simulink model "QD2_IOCheck_2021b"  (R2021b)
settings: Solver=ode2  StartTime=0.0  StopTime=inf  FixedStep=1/1000  RelTol=1e-3  EnableMultiTasking=on
undefined symbols (not defined in the file): HIL, qc_get_step_size
libraries: quarc_library x32, simulink_extras x8, simulink x7
settings Model: DataTypeOverride=Double  MinMaxOverflowLogging=ForceOff  SimulationMode=external  ExtModeTrigElement=1  ExtModeTrigDuration=10000  ExtModeTrigLevel=0.400000  Creator=dmadill  LastModifiedBy=AVRS_ADMIN
settings SolverCC: AlgebraicLoopSolver=TrustRegion  PositivePriorityOrder=on
settings DataIOCC: ReturnWorkspaceOutputs=off
settings DebuggingCC: SFMachineParentedDataDiag=warning  ArithmeticOperatorsInVariantConditions=warning
settings HardwareCC: ProdBitPerLong=64  ProdLargestAtomicInteger=LongLong  ProdLargestAtomicFloat=Double  ProdLongLongMode=on  ProdHWDeviceType=ARM Compatible->ARM 64-bit (LP64)
settings SFSimCC: SimUseLocalCustomCode=off  CustomCodeUndefinedFunction=UseInterfaceOnly
settings RTWCC: Description=QUARC Linux QDrone2 Target Using Toolchain  SystemTargetFile=quarc_linux_qdrone2.tlc  RTWUseLocalCustomCode=off  Toolchain=QUARC linux_qdrone2 | gmake (64-bit Windows)  BuildConfiguration=Faster Runs
settings CodeAppCC: StateflowObjectComments=on
settings STFCustomTargetCC: ConcurrentExecutionCompliant=on  UseToolchainInfoCompliant=on  SystemTargetFile=quarc_linux_qdrone2.tlc
settings GRTTargetCC: TargetLangStandard=C89/C90 (ANSI)  ParMdlRefBuildCompliant=off  CompOptLevelCompliant=off  CombineOutputUpdateFcns=off  MatFileLogging=off  CPPClassGenCompliant=off  GRTInterface=on  ExtMode=on  ExtModeMexFile=quarc_comm  ExtModeMexArgs='-w -d /tmp -uri %u','tcpip://192.168.2.d:17001'
settings ConfigComp: CovMetricSettings=dswe

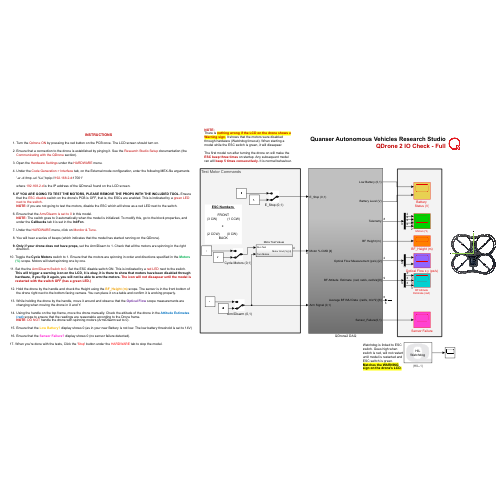
[thumbnail: Simulink's stored preview of the top-level diagram]
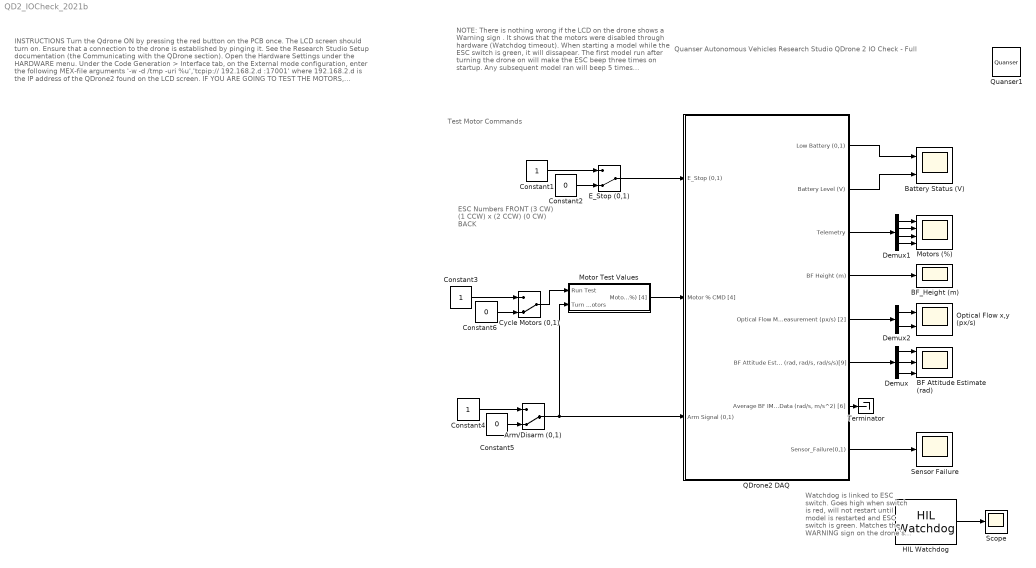
== system QD2_IOCheck_2021b ==
  note: Watchdog is linked to ESC switch. Goes high when switch is red, will not restart until model is restarted and ESC switch is green.
      | Matches the WARNING sign on the drone's LCD.
  note: Test Motor Commands
  note: Quanser Autonomous Vehicles Research Studio
      | QDrone 2 IO Check - Full
  note: ESC Numbers
      |
      | FRONT
      | (3 CW) (1 CCW)
      |
      | x
      |
      | (2 CCW) (0 CW)
      | BACK
  note: INSTRUCTIONS
      |
      | Turn the Qdrone ON by pressing the red button on the PCB once. The LCD screen should turn on.
      |
      | Ensure that a connection to the drone is established by pinging it. See the Research Studio Setup documentation (the Communicating with the QDrone section).
      |
      | Open the Hardware Settings under the HARDWARE menu.
      |
      | Under the Code Generation > Interface tab, on the External mode configuration, enter the following MEX-file arguments
      |
      | '-w -d /tmp -uri %u','tcpip:// 192.168.2.d :17001'
      |
      | where 192.168.2.d is the IP address of the QDrone2 found on the LCD screen.
      |
      | IF YOU ARE GOING TO TEST THE MOTORS, PLEASE REMOVE THE PROPS WITH THE INCLUDED TOOL. Ensure that the ESC disable switch on the drone's PCB is OFF, that is, the ESCs are enabled. This is indicated by a green LED next to the switch .
      | NOTE: if you are not going to test the motors, disable the ESC which will show as a red LED next to the switch.
      |
      | Ensure that the Arm/Disarm is set to 0 in this model.
      | NOTE: The switch goes to 0 automatically when the model is initialized. To modify this, go to the block properties, and under the Callbacks tab it is set in the InitFcn .
      |
      | Under the HARDWARE menu, click on Monitor & Tune .
      |
      | You will hear a series of beeps (which indicates that the model has started running on the QDrone).
      |
      | Only if your drone does not have props, set the Arm/Disarn to 1. Check that all the motors are spinning in the right direction.
      |
      | Toggle the Cycle Motors switch to 1. Ensure that the motors are spinning in order and directions specified in the Motors (%) scope. Motors will start spinning one by one.
      |
      | Set the the Arm/Disarm Switch to 0. Set the ESC disable switch ON. This is indicated by a red LED next to the switch. This will trigger a warning icon on the LCD, it is okay, it is there to show that motors have been disabled through hardware, if you flip it again, you will not be able to arm the motors. The icon will not dissapear until the model is restarted with the switch OFF (has a green LED.)
      |
      | Hold the drone by the handle and check the Height using the BF_Height (m) scope. The sensor is in the front bottom of the drone right next to the bottom facing camera. You can place it on a table and confirm it is working properly.
      |
      | While holding the drone by the handle, move it around and observe that the Optical Flow scope measurements are changing when moving the drone in X and Y.
      |
      | Using the handle on the top frame, move the drone manually. Check the attitude of the drone in the Attitude Estimates (rad) scope to ensure that the readings are reasonable according to the Drone frame.
      | NOTE : DO NOT handle the drone with spinning motors (Arm/Disarm set to 0).
      |
      | Ensure that the Low Battery? display shows 0 (as in your new Battery is not low. The low battery threshold is set to 14V)
      |
      | Ensure that the Sensor Failure? display shows 0 (no sensor failure detected).
      |
      | When you're done with the tests, Click the ' Stop ' button under the HARDWARE tab to stop the model.
  note: NOTE:
      | There is nothing wrong if the LCD on the drone shows a Warning sign . It shows that the motors were disabled through hardware (Watchdog timeout). When starting a model while the ESC switch is green, it will dissapear.
      |
      | The first model run after turning the drone on will make the ESC beep three times on startup. Any subsequent model ran will beep 5 times consecutively. It is normal behaviour.
  Arm/Disarm (0,1) : ManualSwitch  InitFcn=set_param(gcb,'sw','0')  CurrentSetting=0
  "BF Attitude Estimate (rad) " : Scope  NumInputPorts=3
  BF_Height (m) : Scope
  Battery Status (V) : Scope  NumInputPorts=2
  Constant1 : Constant
  Constant2 : Constant  Value=0
  Constant3 : Constant
  Constant4 : Constant
  Constant5 : Constant  Value=0
  Constant6 : Constant  Value=0
  Cycle Motors (0,1) : ManualSwitch  InitFcn=set_param(gcb,'sw','0')  CurrentSetting=0
  Demux : Demux  Outputs=3
  Demux1 : Demux
  Demux2 : Demux  Outputs=2
  E_Stop (0,1) : ManualSwitch  CurrentSetting=0
  HIL Watchdog : quarc_library/Data Acquisition/Generic/Watchdog/HIL Watchdog  object_name=HIL-1  timeout=0.1  sample_time=qc_get_step_size  active=off
      settings: AttributesFormatString=(%<object_name>)  SourceProductName=QUARC Targets
  Motor Test Values : Subsystem
  Motors (%) : Scope  NumInputPorts=4
  Optical Flow x,y (px/s) : Scope  NumInputPorts=2
  QDrone2 DAQ : Subsystem
  Quanser1 : quarc_library/Logos/Quanser
  Scope : Scope
  Sensor Failure : Scope
  Terminator : Terminator
  wires:
  Constant4/1 -> Arm/Disarm (0,1)/1
  Constant5/1 -> Arm/Disarm (0,1)/2
  Constant2/1 -> E_Stop (0,1)/2
  Constant1/1 -> E_Stop (0,1)/1
  E_Stop (0,1)/1 -> QDrone2 DAQ/1(E_Stop (0,1))
  QDrone2 DAQ/6("BF Attitude Estimate (rad, rad/s, rad/s/s)[9]") -> Demux/1
  Demux/1 -> "BF Attitude Estimate (rad) "/1
  Demux/2 -> "BF Attitude Estimate (rad) "/2
  Demux/3 -> "BF Attitude Estimate (rad) "/3
  QDrone2 DAQ/1(Low Battery (0,1)) -> Battery Status (V)/1
  QDrone2 DAQ/2(Battery Level (V)) -> Battery Status (V)/2
  QDrone2 DAQ/8(Sensor_Failure(0,1)) -> Sensor Failure/1
  QDrone2 DAQ/4("BF Height (m) ") -> BF_Height (m)/1
  QDrone2 DAQ/5(Optical Flow Measurement (px/s) [2]) -> Demux2/1
  Demux2/1 -> Optical Flow x,y (px/s)/1
  Demux2/2 -> Optical Flow x,y (px/s)/2
  Motor Test Values/1(Motor Cmd (%) [4]) -> QDrone2 DAQ/2(Motor % CMD [4])
  Arm/Disarm (0,1)/1 -> QDrone2 DAQ/3(Arm Signal (0,1)), Motor Test Values/2(Turn Motors)
  Demux1/3 -> Motors (%)/3
  Demux1/2 -> Motors (%)/2
  Demux1/4 -> Motors (%)/4
  Demux1/1 -> Motors (%)/1
  QDrone2 DAQ/3(Telemetry) -> Demux1/1
  QDrone2 DAQ/7("Average BF IMU Data (rad/s, m/s^2) [6]") -> Terminator/1
  HIL Watchdog/1 -> Scope/1
  Constant6/1 -> Cycle Motors (0,1)/2
  Constant3/1 -> Cycle Motors (0,1)/1
  Cycle Motors (0,1)/1 -> Motor Test Values/1(Run Test)

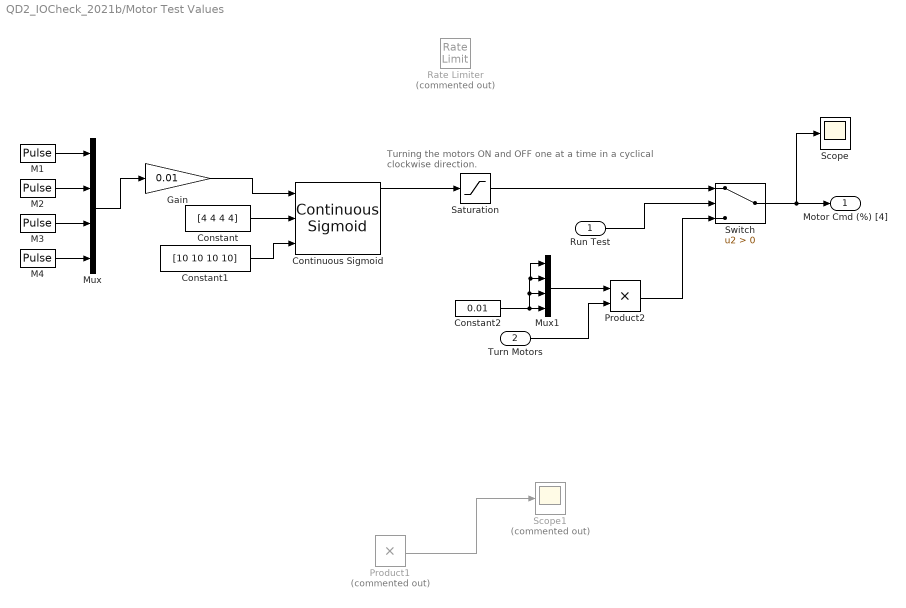
== system QD2_IOCheck_2021b/Motor Test Values ==
  note: Turning the motors ON and OFF one at a time in a cyclical
      | clockwise direction.
  Run Test : Inport
  Turn Motors : Inport  Port=2
  Constant : Constant  Value=[4 4 4 4]
  Constant1 : Constant  Value=[10 10 10 10]
  Constant2 : Constant  Value=0.01
  Continuous Sigmoid : quarc_library/Sources/Sigmoids/Continuous Sigmoid  params_source=External (input ports)  max_velocity=10  max_acceleration=10  initial_position=0  initial_velocity=0  hold_off=0.5  input_sample_time=-1  output_sample_time=qc_get_step_size
      settings: SourceProductName=QUARC Targets
  Gain : Gain  Gain=0.01
  M1 : DiscretePulseGenerator  PulseType=Time based  Period=8  PulseWidth=12.5
  M2 : DiscretePulseGenerator  PulseType=Time based  Period=8  PulseWidth=12.5  PhaseDelay=6
  M3 : DiscretePulseGenerator  PulseType=Time based  Period=8  PulseWidth=12.5  PhaseDelay=2
  M4 : DiscretePulseGenerator  PulseType=Time based  Period=8  PulseWidth=12.5  PhaseDelay=4
  Mux : Mux
  Mux1 : Mux
  Product1 : Product  Commented=on
  Product2 : Product
  Rate Limiter : RateLimiter  Commented=on  RisingSlewLimit=0.1  FallingSlewLimit=-0.1  SampleTimeMode=inherited
  Saturation : Saturate  UpperLimit=0.1  LowerLimit=0
  Scope : Scope
  Scope1 : Scope  Commented=on
  Switch : Switch  Criteria=u2 > Threshold
  Motor Cmd (%) [4] : Outport  VectorParamsAs1DForOutWhenUnconnected=off
  wires:
  M2/1 -> Mux/2
  M3/1 -> Mux/3
  M4/1 -> Mux/4
  M1/1 -> Mux/1
  Continuous Sigmoid/1 -> Saturation/1
  Mux/1 -> Gain/1
  Gain/1 -> Continuous Sigmoid/1
  Constant/1 -> Continuous Sigmoid/2
  Constant1/1 -> Continuous Sigmoid/3
  Product1/1 -> Scope1/1
  Product2/1 -> Switch/3
  Saturation/1 -> Switch/1
  Turn Motors/1 -> Product2/2
  Switch/1 -> Scope/1, Motor Cmd (%) [4]/1
  Run Test/1 -> Switch/2
  Mux1/1 -> Product2/1
  Constant2/1 -> Mux1/1, Mux1/2, Mux1/3, Mux1/4

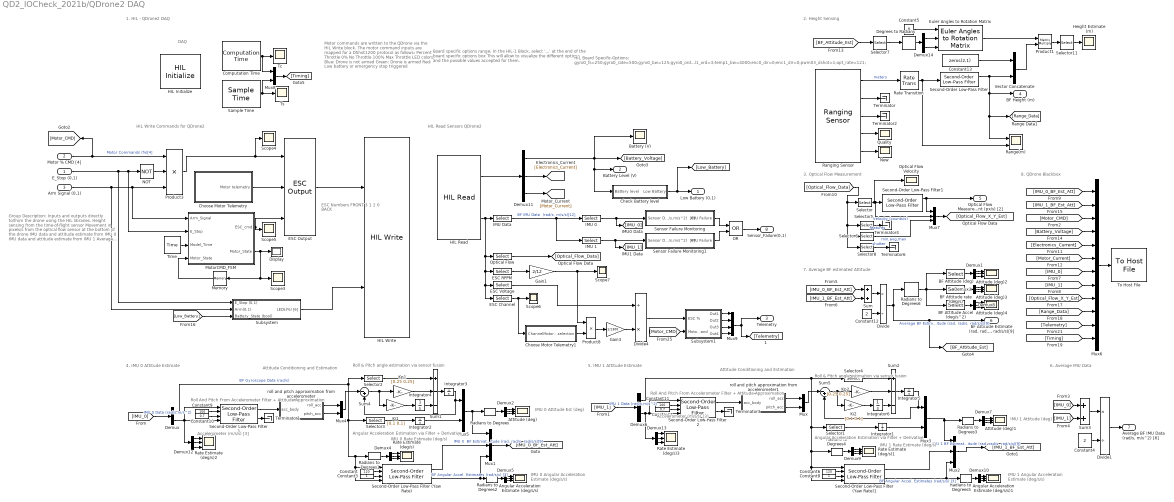
== system QD2_IOCheck_2021b/QDrone2 DAQ ==
  note: 1. HIL - QDrone2 DAQ
  note: HIL Write Commands for QDrone2
  note: ESC Numbers
      |
      | FRONT
      | 3 1
      |
      | 2 0
      | BACK
  note: DAQ
  note: HIL Read Sensors QDrone2
  note: 2. Height Sensing
  note: 3. Optical Flow Measurement
  note: Angular Acceleration Estimation via Filter + Derivative
  note: Roll And Pitch From Accelerometer Filter + Attitude Approximation
  note: Attitude Conditioning and Estimation
  note: 5. IMU 1 Attitude Estimate
  note: IMU 0
      | Rate Estimate (deg/s)
  note: 7. Average BF estimated Attitude
  note: Accelerometer (m/s/s) [3]
  note: Accelerometer (m/s/s) [3]
  note: Roll & Pitch angle estimation via sensor fusion
  note: IMU 1
      | Angular Acceleration
      | Estimate (deg/s/s)
  note: Roll And Pitch From Accelerometer Filter + Attitude Approximation
  note: IMU 1
      | Attitude (deg)
  note: IMU 0
      | Angular Acceleration
      | Estimate (deg/s/s)
  note: Roll & Pitch angle estimation via sensor fusion
  note: Attitude Conditioning and Estimation
  note: 4. IMU 0 Attitude Estimate
  note: IMU 0
      | Attitude Est (deg)
  note: 8. QDrone Blackbox
  note: Angular Acceleration Estimation via Filter + Derivative
  note: 6. Average IMU Data
  note: IMU 1
      | Rate Estimate (deg/s)
  note: Motor commands are written to the QDrone via the HIL Write block. The motor command inputs are mapped for a DShot1200 protocol as follows:
      |
      | Percent Throttle
      | 0% No Throttle
      | 100% Max Throttle
      |
      | LED colors:
      | Blue: Drone is not armed
      | Green: Drone is armed
      | Red: Low battery or emergency stop triggered
  note: Board specific options range:
      |
      | In the HIL-1 Block,
      | select '...' at the end of the board specific options box
      | This will allow to visualize the different options
      | and the possible values accepted for them.
  note: HIL Board Specific-Options:
      | gyro0_fs=250;gyro0_rate=500;gyro0_bw=125;gyro0_ord=3;accel0_fs=16;accel0_rate=1000;accel0_bw=400;accel0_ord=3;temp0_bw=4000;gyro1_fs=250;gyro1_rate=500;gyro1_bw=125;gyro1_ord=3;accel1_fs=16;accel1_rate=1000;accel1_bw=400;accel1_ord=3;temp1_bw=4000;enc0_dir=0;enc1_dir=0;pwm03_dshot=1;opt_rate=121;
  note: Group Description:
      |
      | Inputs and outputs directly to/from the drone using the HIL libraries.
      | Height sensing from the time-of-flight sensor
      | Movement in pixels/s from the optical flow sensor at the bottom of the drone
      | IMU data and attitude estimate from IMU 0
      | IMU data and attitude estimate from IMU 1
      | Average of both IMU outputs
      | Average body frame attitude from IMU data
      | Blackbox saving all relevant values
  E_Stop (0,1) : Inport
  Motor % CMD [4] : Inport  Port=2
  Arm Signal (0,1) : Inport  Port=3
  Angular Acceleration Estimate (deg/s/s) : Scope  NumInputPorts=3
  Angular Acceleration Estimate (deg/s/s)1 : Scope  NumInputPorts=3
  Attitude (deg){,1..4} (5 alike) : Scope  NumInputPorts=3
  BF Attitude (deg) : Selector  InputPortWidth=9  IndexOptions=Index vector (dialog)  Indices=[1:3]  OutputSizes=1
  BF Attitude Accel (deg/s^2) : Selector  InputPortWidth=9  IndexOptions=Index vector (dialog)  Indices=[7:9]  OutputSizes=1
  BF Attitude rate (deg/s) : Selector  InputPortWidth=9  IndexOptions=Index vector (dialog)  Indices=[4:6]  OutputSizes=1
  Battery (V) : Scope
  Check Battery level : Subsystem
  Choose Motor Telemetry : Subsystem
  Choose Motor Telemetry1 : Subsystem
  Computation Time : quarc_library/Sources/Time/Computation Time  sample_time=qc_get_step_size  use_model=on  use_cpu_time=off
  Constant : Constant  Value=120
  Constant10 : Constant  Value=0.7
  Constant11 : Constant  Value=100
  Constant12 : Constant  Value=2
  Constant13 : Constant  Value=zeros(2,1)
  Constant3 : Constant
  Constant4 : Constant  Value=2
  Constant5 : Constant  Value=0
  Constant6 : Constant  Value=120
  Constant7 : Constant  Value=0.7
  Constant8 : Constant
  Constant9 : Constant  Value=100
  Degrees to Radians : simulink_extras/Transformations/Degrees to Radians
  Demux : Demux  Outputs=[3,3]
  Demux{1..5,7..13} (12 alike) : Demux  Outputs=3
  Demux14 : Demux  Outputs=2
  Demux6 : Demux  Outputs=[3,3]
  Display : Display
  Divide : Product  Inputs=*/
  Divide1 : Product  Inputs=*/
  Divide4 : Product  Inputs=/*
  ESC Channel : Selector  InputPortWidth=22  IndexOptions=Index vector (dialog)  Indices=[22]  OutputSizes=1
  ESC Output : quarc_library/Data Acquisition/Generic/Transformations/ESC Output  protocol=DShot (raw)
      settings: AttributesFormatString=%<protocol>  SourceProductName=QUARC Targets
  ESC RPPM : Selector  InputPortWidth=22  IndexOptions=Index vector (dialog)  Indices=[20]  OutputSizes=1
  ESC Voltage : Selector  InputPortWidth=22  IndexOptions=Index vector (dialog)  Indices=[21]  OutputSizes=1
  Euler Angles to Rotation Matrix : quarc_library/Math Operations/Matrices/Euler Angles to Rotation Matrix  menu_order=Relative Z-X-Y
      settings: SourceProductName=QUARC Targets
  Gain1 : Gain  Gain=2/12
  Gain3 : Gain  Gain=1/1300
  HIL Initialize : quarc_library/Data Acquisition/Generic/Configuration/HIL Initialize  object_name=HIL-1  board_type=qdrone2  board_number=0  board_options=gyro0_fs=250;gyro0_rate=500;gyro0_bw=125;gyro0_ord=3;accel0_fs=16;accel0_rate=1000;accel0_bw=400;accel0_ord=3;temp0_bw=4000;gyro1_fs=250;gyro1_rate=500;gyro1_bw=125;gyro1_ord=3;accel1_fs=16;accel1_rate=1000;accel1_bw=400;accel1_ord=3;temp1_bw=4000;enc0_dir=0;enc1_dir=0;pwm03_dshot=1;opt_rate=121;  exclusive=off  active=on  hardware_clocks=[]  clock_modes=[]  initial_clock_frequencies=[]  set_clock_params_at_start=off  set_clock_params_at_switch_in=off  set_clock_frequencies_at_start=off  set_clock_frequencies_at_switch_in=off  analog_input_channels=[0:3]  analog_input_configurations=[]  analog_input_maximums=[3.3]  analog_input_minimums=[0]  set_analog_input_params_at_start=off  set_analog_input_params_at_switch_in=off  analog_output_channels=[]  analog_output_maximums=[]  analog_output_minimums=[]  initial_analog_outputs=[]  final_analog_outputs=[]  watchdog_analog_outputs=[]  set_analog_output_params_at_start=off  set_analog_output_params_at_switch_in=off  set_analog_outputs_at_start=off  set_analog_outputs_at_switch_in=off  set_analog_outputs_at_terminate=off  set_analog_outputs_at_switch_out=off  set_analog_outputs_on_watchdog=off  digital_input_channels=[0:5]  digital_output_channels=[6:11]  digital_output_configuration=[]  initial_digital_outputs=[0]  final_digital_outputs=[0]  watchdog_digital_outputs=[0 0 0 0 0 0]  set_digital_output_params_at_start=off  set_digital_output_params_at_switch_in=off  set_digital_outputs_at_start=on  set_digital_outputs_at_switch_in=off  set_digital_outputs_at_terminate=on  set_digital_outputs_at_switch_out=off  set_digital_outputs_on_watchdog=off  encoder_channels=[0:1]  quadrature=[4]  encoder_filter_frequency=100e6/1  initial_encoder_counts=[0]  set_encoder_params_at_start=on  set_encoder_params_at_switch_in=off  set_encoder_counts_at_start=on  set_encoder_counts_at_switch_in=off  pwm_channels=[0:5]  pwm_modes=[6 6 6 6 0 0]  pwm_frequency=1.2e6  pwm_configuration=[0]  pwm_alignment=[0]  pwm_polarity=[1]  pwm_leading_deadband=[]  pwm_trailing_deadband=[]  initial_pwm_outputs=[0]  final_pwm_outputs=[0]  watchdog_pwm_outputs=[0]  set_pwm_params_at_start=on  set_pwm_params_at_switch_in=off  set_pwm_outputs_at_start=on  set_pwm_outputs_at_switch_in=off  set_pwm_outputs_at_terminate=on  set_pwm_outputs_at_switch_out=off  set_pwm_outputs_on_watchdog=on  other_output_channels=[]  initial_other_outputs=[]  final_other_outputs=[]  watchdog_other_outputs=[]  set_other_outputs_at_start=on  set_other_outputs_at_switch_in=off  set_other_outputs_at_terminate=on  set_other_outputs_at_switch_out=off  set_other_outputs_on_watchdog=off
  HIL Read : quarc_library/Data Acquisition/Generic/Immediate I//O/HIL Read  object_name=HIL-1  analog_channels=[3 1:2]  encoder_channels=[]  digital_channels=[]  other_channels=[3000:3002 4000:4002 3003:3005 4003:4005 17000:17006 17008:17009 17007]  sample_time=qc_get_step_size  active=on  vector_output=on  data_type_mode=Inherit via back propagation  encoder_data_type=double  digital_data_type=boolean
  HIL Write : quarc_library/Data Acquisition/Generic/Immediate I//O/HIL Write  object_name=HIL-1  analog_channels=[]  pwm_channels=[0:3]  digital_channels=[6:11]  other_channels=[]  sample_time=-1  active=off  vector_input=on
  Height Estimate (m) : Scope
  IMU 0 : Selector  InputPortWidth=12  IndexOptions=Index vector (dialog)  Indices=[1:6]  OutputSizes=1
  IMU 1 : Selector  InputPortWidth=12  IndexOptions=Index vector (dialog)  Indices=[7:12]  OutputSizes=1
  IMU Data : Selector  InputPortWidth=22  IndexOptions=Index vector (dialog)  Indices=[1:12]  OutputSizes=1
  Integrator{1..6} (6 alike) : Integrator
  Ki1 : Gain  Gain=[0.1 0.1]
  Ki2 : Gain  Gain=[0.1 0.1]
  Kp1 : Gain  Gain=[0.25 0.25]
  Kp2 : Gain  Gain=[0.25 0.25]
  Memory : Memory
  MotorCMD_FSM : MATLAB Function  TreatAsAtomicUnit=on
  Mux{,3..5,8} (5 alike) : Mux  Inputs=2
  Mux1 : Mux  Inputs=3
  Mux2 : Mux  Inputs=3
  Mux6 : Mux  Inputs=12
  Mux7 : Mux  Inputs=3
  Mux9 : Mux
  NOT : Logic  Operator=NOT  IconShape=distinctive  AllPortsSameDT=off  OutDataTypeStr=boolean
  New : Scope
  OR : Logic  Operator=OR  AllPortsSameDT=off  OutDataTypeStr=boolean
  Optical Flow : Selector  InputPortWidth=22  IndexOptions=Index vector (dialog)  Indices=[13:19]  OutputSizes=1
  Optical Flow Velocity : Scope
  Product1 : Product  Multiplication=Matrix(*)
  Product3 : Product  Inputs=3
  Product8 : Product
  Quality : Scope
  Radians to Degrees{,1..6} (7 alike) : simulink_extras/Transformations/Radians to Degrees
  Range(m) : Scope  NumInputPorts=2
  Ranging Sensor : quarc_library/Devices/Third-Party/Sensors/Ranging Sensor  sensor_type=VL53L1X Time-of-flight  uri=i2c-cpu://localhost:0?address='0x29',baud='400000',memsize='512'  ranging_distance=Long  timing_budget=0.033  measurement_period=0.040  output_mode=Fixed-size output  samples_per_revolution=1300  max_distance=0.050  max_angle=5  sample_time=qc_get_step_size * ceil(1/121/ qc_get_step_size)  show_versions=off  active=on
      settings: SourceProductName=QUARC Targets
  Rate Estimate (deg/s){,1..3} (4 alike) : Scope  NumInputPorts=3
  Rate Transition : RateTransition
  Sample Time : quarc_library/Sources/Time/Sample Time  Priority=-99  sample_time=qc_get_step_size
  Scope{3..7} (5 alike) : Scope
  Second-Order Low-Pass Filter : quarc_library/Continuous/Second-Order Low-Pass Filter  params_source=Internal (dialog parameters)  input_width=100  input_zeta=0.7  input_init=0
  Second-Order Low-Pass Filter (Yaw Rate) : quarc_library/Continuous/Second-Order Low-Pass Filter  params_source=External (input ports)  input_width=200  input_zeta=1  input_init=0
  Second-Order Low-Pass Filter (Yaw Rate)1 : quarc_library/Continuous/Second-Order Low-Pass Filter  params_source=External (input ports)  input_width=200  input_zeta=1  input_init=0
  Second-Order Low-Pass Filter 1 : quarc_library/Continuous/Second-Order Low-Pass Filter  params_source=External (input ports)  input_width=50  input_zeta=1  input_init=0
  Second-Order Low-Pass Filter 2 : quarc_library/Continuous/Second-Order Low-Pass Filter  params_source=External (input ports)  input_width=50  input_zeta=1  input_init=0
  Second-Order Low-Pass Filter1 : quarc_library/Continuous/Second-Order Low-Pass Filter  params_source=Internal (dialog parameters)  input_width=45  input_zeta=1.5  input_init=0
  Selector : Selector  InputPortWidth=7  IndexOptions=Index vector (dialog)  Indices=[1 2]  OutputSizes=1
  Selector1 : Selector  InputPortWidth=3  IndexOptions=Index vector (dialog)  Indices=[3]  OutputSizes=1
  Selector11 : Selector  InputPortWidth=3  IndexOptions=Index vector (dialog)  Indices=[3]  OutputSizes=1
  Selector2 : Selector  InputPortWidth=3  IndexOptions=Index vector (dialog)  Indices=[1,2]  OutputSizes=1
  Selector3 : Selector  InputPortWidth=3  IndexOptions=Index vector (dialog)  Indices=[3]  OutputSizes=1
  Selector4 : Selector  InputPortWidth=3  IndexOptions=Index vector (dialog)  Indices=[1,2]  OutputSizes=1
  Selector5 : Selector  InputPortWidth=7  IndexOptions=Index vector (dialog)  Indices=[3]  OutputSizes=1
  Selector6 : Selector  InputPortWidth=7  IndexOptions=Index vector (dialog)  Indices=[4 5 6]  OutputSizes=1
  Selector7 : Selector  InputPortWidth=9  IndexOptions=Index vector (dialog)  Indices=[1,2]  OutputSizes=1
  Selector8 : Selector  InputPortWidth=7  IndexOptions=Index vector (dialog)  Indices=[7]  OutputSizes=1
  Sensor Failure Monitoring : Subsystem
  Sensor Failure Monitoring1 : Subsystem
  Subsystem : Subsystem
  Subsystem1 : Subsystem
  Sum : Sum
  Sum1 : Sum  Inputs=+--
  Sum2 : Sum  Inputs=+--
  Sum3 : Sum
  Sum4 : Sum  Inputs=|-+
  Sum5 : Sum  Inputs=|-+
  Tc : Scope
  Terminator{,1..4,6} (6 alike) : Terminator
  Time : quarc_library/Sources/Time/Time  time_source=Wall clock  sample_time=qc_get_step_size
  To Host File : quarc_library/Sinks/To Host/To Host File  file_name=saved_data/%m/QDrone2_%{date}_%{time}.mat  variable_name=QDrone_data  decimation=1  sample_time=-1  file_format=MAT-file v.4  options=No header or footer  append=off  final_file_name=saved_data/QDrone2_IO_Check_2021b/QDrone2_10-Apr-2023_14-56-11.mat  bitrate=2000000
  Ts : Scope
  Vector Concatenate : Concatenate
  roll and pitch approximation from accelerometer : MATLAB Function  TreatAsAtomicUnit=on
  roll and pitch approximation from accelerometer1 : MATLAB Function  TreatAsAtomicUnit=on
  Low Battery (0,1) : Outport
  Battery Level (V) : Outport  Port=2
  Telemetry : Outport  Port=3
  "BF Height (m) " : Outport  Port=4
  Optical Flow Measurement (px/s) [2] : Outport  Port=5
  "BF Attitude Estimate (rad, rad/s, rad/s/s)[9]" : Outport  Port=6
  "Average BF IMU Data (rad/s, m/s^2) [6]" : Outport  Port=7
  Sensor_Failure(0,1) : Outport  Port=8
  wires:
  Subsystem/1(LEDs(%) [6]) -> HIL Write/2
  [Low_Battery] -> Subsystem/3(Battery_State (bool))
  Arm Signal (0,1)/1 -> Product3/3, MotorCMD_FSM/1(Arm_Signal), Subsystem/2("Arm(0,1) ")
  NOT/1 -> Product3/2
  Motor % CMD [4]/1 -> [Motor_CMD], Product3/1  "Motor Commands (%)[4]"
  E_Stop (0,1)/1 -> Subsystem/1(E_Stop (0,1)), MotorCMD_FSM/2(E_Stop), NOT/1
  Time/1 -> MotorCMD_FSM/3(Model_Time)
  MotorCMD_FSM/2(Motor_State) -> Scope3/1, Memory/1, Display/1
  Memory/1 -> MotorCMD_FSM/4("Motor_State ")
  Choose Motor Telemetry/1(Motor telemetry) -> ESC Output/2
  ESC Output/1 -> HIL Write/1
  MotorCMD_FSM/1(ESC_cmd) -> ESC Output/3, Scope5/1
  Product3/1 -> Scope4/1, ESC Output/1
  OR/1 -> Sensor_Failure(0,1)/1
  Gain3/1 -> Divide4/2
  [Motor_CMD] -> Subsystem1/2(Motor command)
  ESC Channel/1 -> Scope6/1, Choose Motor Telemetry1/1(Channel)
  HIL Read/2 -> IMU Data/1, ESC RPPM/1, ESC Voltage/1, ESC Channel/1, Optical Flow/1
  ESC RPPM/1 -> Gain1/1
  Gain1/1 -> Product8/1, Scope7/1
  Product8/1 -> Gain3/1
  ESC Voltage/1 -> Divide4/1
  Choose Motor Telemetry1/1(Motor selection) -> Product8/2
  Divide4/1 -> Subsystem1/1(ESC %)
  Check Battery level/1(Low Battery) -> [Low_Battery], Low Battery (0,1)/1
  IMU 1/1 -> [IMU_1], Sensor Failure Monitoring1/1(Sensor Data (rad/s,m/s^2)  [6])
  Sensor Failure Monitoring/1(IMU Failure) -> OR/1
  IMU 0/1 -> [IMU_0], Sensor Failure Monitoring/1(Sensor Data (rad/s,m/s^2)  [6])
  Demux11/1 -> Battery Level (V)/1, Check Battery level/1(Battery level), [Battery_Voltage], Battery (V)/1
  HIL Read/1 -> Demux11/1
  Demux11/3 -> [Motor_Current]
  Demux11/2 -> [Electronics_Current]
  Mux9/1 -> Telemetry/1, [Telemetry]
  Sensor Failure Monitoring1/1(IMU Failure) -> OR/2
  Subsystem1/4(Out4) -> Mux9/4
  IMU Data/1 -> IMU 1/1, IMU 0/1  "BF IMU Data  (rad/s, m/s/s)[12]"
  Subsystem1/2(Out2) -> Mux9/2
  Subsystem1/1(Out1) -> Mux9/1
  Subsystem1/3(Out3) -> Mux9/3
  Optical Flow/1 -> [Optical_Flow_Data]
  Ranging Sensor/2 -> Terminator/1
  Rate Transition/1 -> Range(m)/2, Second-Order Low-Pass Filter/1
  Constant5/1 -> Euler Angles to Rotation Matrix/1
  Selector7/1 -> Degrees to Radians/1
  Euler Angles to Rotation Matrix/1 -> Product1/1
  Ranging Sensor/3 -> Terminator2/1
  Second-Order Low-Pass Filter1/1 -> Optical Flow Measurement (px/s) [2]/1, Mux7/1
  Vector Concatenate/1 -> Product1/2
  Second-Order Low-Pass Filter/1 -> [Range_Data], Range(m)/1, "BF Height (m) "/1, Vector Concatenate/2
  Ranging Sensor/4 -> Quality/1
  Ranging Sensor/1 -> Rate Transition/1  "meters"
  Demux14/2 -> Euler Angles to Rotation Matrix/3
  Product1/1 -> Selector11/1
  Degrees to Radians/1 -> Demux14/1
  Selector11/1 -> Height Estimate (m)/1
  [Optical_Flow_Data] -> Selector/1, Selector8/1, Selector6/1, Selector5/1
  Ranging Sensor/5 -> New/1
  Demux14/1 -> Euler Angles to Rotation Matrix/2
  Constant13/1 -> Vector Concatenate/1
  [BF_Attitude_Est] -> Selector7/1
  BF Attitude rate (deg/s)/1 -> Demux3/1
  Demux12/3 -> Rate Estimate (deg/s)2/3
  Radians to Degrees2/1 -> Demux5/1
  Demux1/1 -> Attitude (deg)2/1
  [IMU_0] -> Sum3/1
  Demux12/1 -> Rate Estimate (deg/s)2/1
  Sum5/1 -> Kp2/1, Ki2/1
  Sum/1 -> Divide/1
  [IMU_1_BF_Est_Att] -> Mux6/2
  [Motor_Current] -> Mux6/6
  [Battery_Voltage] -> Mux6/4
  [IMU_0] -> Mux6/7
  Second-Order Low-Pass Filter (Yaw Rate)1/2 -> Radians to Degrees5/1, Mux2/3  "BF Angular Accel. Estimates (rad/s/s) [3]"
  Sum3/1 -> Divide1/1
  Ki1/1 -> Integrator4/1
  [IMU_0_BF_Est_Att] -> Mux6/1
  Mux6/1 -> To Host File/1
  Integrator4/1 -> Sum1/3
  Integrator3/1 -> Sum4/2, Mux5/1
  Demux7/2 -> Attitude (deg)1/2
  [Electronics_Current] -> Mux6/5
  Demux8/3 -> Attitude (deg)4/3
  Divide1/1 -> "Average BF IMU Data (rad/s, m/s^2) [6]"/1
  Sum4/1 -> Kp1/1, Ki1/1
  Demux3/1 -> Attitude (deg)3/1
  [IMU_0] -> Demux/1  "IMU 0 Data (rad/s,m/s^2)"
  Mux4/1 -> Sum4/1
  Sum2/1 -> Integrator5/1
  [IMU_1_BF_Est_Att] -> Sum/2
  [IMU_0_BF_Est_Att] -> Sum/1
  BF Attitude (deg)/1 -> Demux1/1
  Demux1/2 -> Attitude (deg)2/2
  BF Attitude Accel (deg/s^2)/1 -> Demux8/1
  Demux/1 -> Radians to Degrees1/1, Second-Order Low-Pass Filter (Yaw Rate)/4, Second-Order Low-Pass Filter (Yaw Rate)/1, Selector3/1, Selector2/1  "BF Gyroscope Data (rad/s)"
  Constant11/1 -> Second-Order Low-Pass Filter 2/2
  Constant4/1 -> Divide1/2
  Demux5/2 -> Angular Acceleration Estimate (deg/s/s)/2
  Demux5/1 -> Angular Acceleration Estimate (deg/s/s)/1
  Second-Order Low-Pass Filter 1/1 -> roll and pitch approximation from accelerometer/1(acc_body)
  Demux4/1 -> Rate Estimate (deg/s)/1
  Radians to Degrees5/1 -> Demux10/1
  Demux5/3 -> Angular Acceleration Estimate (deg/s/s)/3
  Integrator6/1 -> Sum2/3
  Demux2/1 -> Attitude (deg)/1
  Selector1/1 -> Integrator1/1
  roll and pitch approximation from accelerometer/1(roll_acc) -> Mux4/1
  Mux/1 -> Sum5/1
  Demux1/3 -> Attitude (deg)2/3
  Sum1/1 -> Integrator3/1
  Selector4/1 -> Sum2/1
  Divide/1 -> Radians to Degrees6/1, [BF_Attitude_Est], "BF Attitude Estimate (rad, rad/s, rad/s/s)[9]"/1  "Average BF Estimated Attitude (rad, rad/s, rad/s/s)[9]"
  Demux2/2 -> Attitude (deg)/2
  roll and pitch approximation from accelerometer1/1(roll_acc) -> Mux/1
  Kp1/1 -> Sum1/2
  Mux3/1 -> Radians to Degrees3/1, Mux2/1
  Radians to Degrees3/1 -> Demux7/1
  Constant/1 -> Second-Order Low-Pass Filter (Yaw Rate)/2
  Demux8/2 -> Attitude (deg)4/2
  Mux5/1 -> Mux1/1, Radians to Degrees/1
  Demux10/1 -> Angular Acceleration Estimate (deg/s/s)1/1
  Mux1/1 -> [IMU_0_BF_Est_Att]  "IMU 0  BF Estimated Attitude (rad, rad/s, rad/s/s)[9]"
  Ki2/1 -> Integrator6/1
  Demux12/2 -> Rate Estimate (deg/s)2/2
  [IMU_1] -> Demux6/1  "IMU 1 Data (rad/s,m/s^2)"
  Demux3/3 -> Attitude (deg)3/3
  Constant6/1 -> Second-Order Low-Pass Filter (Yaw Rate)1/2
  Demux9/3 -> Rate Estimate (deg/s)1/3
  [IMU_1] -> Sum3/2
  roll and pitch approximation from accelerometer1/2(pitch_acc) -> Mux/2
  Demux10/2 -> Angular Acceleration Estimate (deg/s/s)1/2
  Demux/2 -> Demux12/1, Second-Order Low-Pass Filter 1/1, Second-Order Low-Pass Filter 1/4
  Radians to Degrees4/1 -> Demux9/1
  Demux6/1 -> Selector4/1, Second-Order Low-Pass Filter (Yaw Rate)1/4, Second-Order Low-Pass Filter (Yaw Rate)1/1, Radians to Degrees4/1, Selector1/1
  Radians to Degrees1/1 -> Demux4/1
  Integrator5/1 -> Sum5/2, Mux3/1
  Second-Order Low-Pass Filter (Yaw Rate)/2 -> Mux1/3, Radians to Degrees2/1  "BF Angular Accel. Estimates (rad/s/s) [3]"
  Radians to Degrees/1 -> Demux2/1
  Demux4/2 -> Rate Estimate (deg/s)/2
  Demux9/2 -> Rate Estimate (deg/s)1/2
  Selector2/1 -> Sum1/1
  Kp2/1 -> Sum2/2
  Second-Order Low-Pass Filter 2/1 -> roll and pitch approximation from accelerometer1/1(acc_body)
  Second-Order Low-Pass Filter (Yaw Rate)/1 -> Mux1/2
  Constant9/1 -> Second-Order Low-Pass Filter 1/2
  Demux2/3 -> Attitude (deg)/3
  Demux10/3 -> Angular Acceleration Estimate (deg/s/s)1/3
  Demux4/3 -> Rate Estimate (deg/s)/3
  [Range_Data] -> Mux6/10
  Demux3/2 -> Attitude (deg)3/2
  Demux7/3 -> Attitude (deg)1/3
  Integrator2/1 -> Mux5/2
  Constant8/1 -> Second-Order Low-Pass Filter (Yaw Rate)1/3
  roll and pitch approximation from accelerometer/2(pitch_acc) -> Mux4/2
  Constant10/1 -> Second-Order Low-Pass Filter 1/3
  Demux9/1 -> Rate Estimate (deg/s)1/1
  Demux7/1 -> Attitude (deg)1/1
  Integrator1/1 -> Mux3/2
  Second-Order Low-Pass Filter 2/2 -> Terminator3/1
  [Optical_Flow_X_Y_Est] -> Mux6/9
  Constant3/1 -> Second-Order Low-Pass Filter (Yaw Rate)/3
  Constant7/1 -> Second-Order Low-Pass Filter 2/3
  Mux2/1 -> [IMU_1_BF_Est_Att]  "IMU 1 BF Estimated Attitude (rad, rad/s, rad/s/s)[9]"
  Second-Order Low-Pass Filter 1/2 -> Terminator1/1
  Demux8/1 -> Attitude (deg)4/1
  [IMU_1] -> Mux6/8
  Radians to Degrees6/1 -> BF Attitude (deg)/1, BF Attitude rate (deg/s)/1, BF Attitude Accel (deg/s^2)/1
  Selector3/1 -> Integrator2/1
  Constant12/1 -> Divide/2
  Second-Order Low-Pass Filter (Yaw Rate)1/1 -> Mux2/2
  [Motor_CMD] -> Mux6/3
  Sample Time/1 -> Mux8/2, Ts/1
  Computation Time/1 -> Mux8/1, Tc/1
  Selector/1 -> Optical Flow Velocity/1, Mux7/2, Second-Order Low-Pass Filter1/1  "Velocity (counts/s)"
  Demux13/1 -> Rate Estimate (deg/s)3/1
  Demux13/2 -> Rate Estimate (deg/s)3/2
  Demux6/2 -> Demux13/1, Second-Order Low-Pass Filter 2/1, Second-Order Low-Pass Filter 2/4
  Demux13/3 -> Rate Estimate (deg/s)3/3
  Selector5/1 -> Terminator4/1  "features"
  Selector6/1 -> Mux7/3  "min,avg,max"
  Selector8/1 -> Terminator6/1  "shutter"
  Mux7/1 -> [Optical_Flow_X_Y_Est]
  Mux8/1 -> [Timing]
  [Timing] -> Mux6/12
  [Telemetry] -> Mux6/11

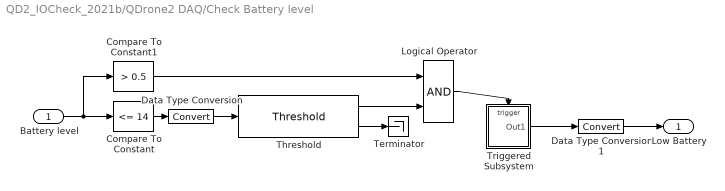
== system QD2_IOCheck_2021b/QDrone2 DAQ/Check Battery level ==
  Battery level : Inport
  Compare To Constant : simulink/Logic and Bit Operations/Compare To Constant  relop=<=  const=14  OutDataTypeStr=boolean
  Compare To Constant1 : simulink/Logic and Bit Operations/Compare To Constant  relop=>  const=0.5  OutDataTypeStr=boolean
  Data Type Conversion : DataTypeConversion
  Data Type Conversion1 : DataTypeConversion
  Logical Operator : Logic  AllPortsSameDT=off  OutDataTypeStr=boolean
  Terminator : Terminator
  Threshold : quarc_library/Discontinuities/Threshold  operator=>=  param_src=Specify via dialog  threshold=0.5  duration=0.3
      settings: SourceProductName=QUARC Targets
  Triggered Subsystem : Subsystem  TreatAsAtomicUnit=on
  Low Battery : Outport  VectorParamsAs1DForOutWhenUnconnected=off
  wires:
  Threshold/2 -> Terminator/1
  Battery level/1 -> Compare To Constant1/1, Compare To Constant/1
  Threshold/1 -> Logical Operator/2
  Logical Operator/1 -> Triggered Subsystem/Trigger
  Compare To Constant1/1 -> Logical Operator/1
  Compare To Constant/1 -> Data Type Conversion/1
  Data Type Conversion/1 -> Threshold/1
  Data Type Conversion1/1 -> Low Battery/1
  Triggered Subsystem/1(Out1) -> Data Type Conversion1/1

== system QD2_IOCheck_2021b/QDrone2 DAQ/Choose Motor Telemetry ==
  Bias1 : Bias  Bias=0:3
  Constant : Constant  Value=[0 0 0 0; 0 0 0 1; 0 0 0 0; 0 0 1 0; 0 0 0 0; 0 1 0 0; 0 0 0 0; 1 0 0 0]
  Counter Free-Running : simulink/Sources/Counter Free-Running  NumBits=3  tsamp=-1
  Gain : Gain  Gain=.7
  Selector : Selector  NumberOfDimensions=2  IndexMode=Zero-based  InputPortWidth=3  IndexOptions=Index vector (port),Select all  Indices=[1 3],1  OutputSizes=1,1
  Telemetry : Scope
  Motor telemetry : Outport
  wires:
  Gain/1 -> Bias1/1
  Bias1/1 -> Telemetry/1
  Constant/1 -> Selector/1
  Counter Free-Running/1 -> Selector/2
  Selector/1 -> Motor telemetry/1, Gain/1

== system QD2_IOCheck_2021b/QDrone2 DAQ/Choose Motor Telemetry1 ==
  Channel : Inport
  Constant1 : Constant  Value=[1 0 0 0]
  Constant2 : Constant  Value=[0 1 0 0]
  Constant3 : Constant  Value=[0 0 1 0]
  Constant4 : Constant  Value=[0 0 0 1]
  Multiport Switch : MultiPortSwitch  DataPortOrder=Zero-based contiguous  Inputs=4  zeroidx=on
  Motor selection : Outport
  wires:
  Multiport Switch/1 -> Motor selection/1
  Constant4/1 -> Multiport Switch/5
  Constant3/1 -> Multiport Switch/4
  Constant1/1 -> Multiport Switch/2
  Constant2/1 -> Multiport Switch/3
  Channel/1 -> Multiport Switch/1

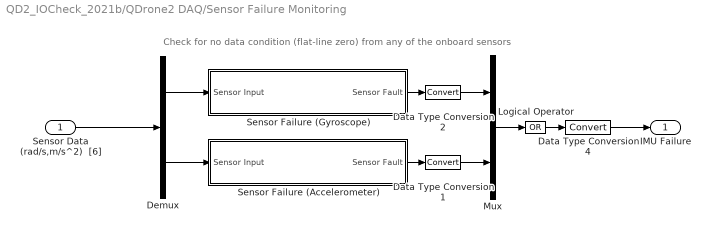
== system QD2_IOCheck_2021b/QDrone2 DAQ/Sensor Failure Monitoring ==
  note: Check for no data condition (flat-line zero) from any of the onboard sensors
  Sensor Data (rad/s,m/s^2)  [6] : Inport
  Data Type Conversion1 : DataTypeConversion
  Data Type Conversion2 : DataTypeConversion
  Data Type Conversion4 : DataTypeConversion
  Demux : Demux  Outputs=[3 3]
  Logical Operator : Logic  Operator=OR  Inputs=1  AllPortsSameDT=off  OutDataTypeStr=boolean
  Mux : Mux  Inputs=2
  Sensor Failure (Accelerometer) : Subsystem
  Sensor Failure (Gyroscope) : Subsystem
  IMU Failure : Outport  VectorParamsAs1DForOutWhenUnconnected=off
  wires:
  Data Type Conversion4/1 -> IMU Failure/1
  Logical Operator/1 -> Data Type Conversion4/1
  Demux/1 -> Sensor Failure (Gyroscope)/1(Sensor Input)
  Data Type Conversion1/1 -> Mux/2
  Data Type Conversion2/1 -> Mux/1
  Mux/1 -> Logical Operator/1
  Sensor Failure (Accelerometer)/1(Sensor Fault) -> Data Type Conversion1/1
  Sensor Failure (Gyroscope)/1(Sensor Fault) -> Data Type Conversion2/1
  Demux/2 -> Sensor Failure (Accelerometer)/1(Sensor Input)
  Sensor Data (rad/s,m/s^2)  [6]/1 -> Demux/1

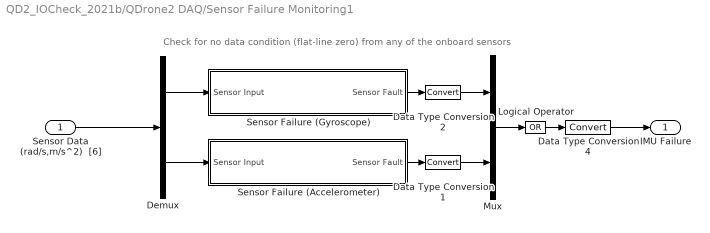
== system QD2_IOCheck_2021b/QDrone2 DAQ/Sensor Failure Monitoring1 ==
  note: Check for no data condition (flat-line zero) from any of the onboard sensors
  Sensor Data (rad/s,m/s^2)  [6] : Inport
  Data Type Conversion1 : DataTypeConversion
  Data Type Conversion2 : DataTypeConversion
  Data Type Conversion4 : DataTypeConversion
  Demux : Demux  Outputs=[3 3]
  Logical Operator : Logic  Operator=OR  Inputs=1  AllPortsSameDT=off  OutDataTypeStr=boolean
  Mux : Mux  Inputs=2
  Sensor Failure (Accelerometer) : Subsystem
  Sensor Failure (Gyroscope) : Subsystem
  IMU Failure : Outport  VectorParamsAs1DForOutWhenUnconnected=off
  wires:
  Sensor Data (rad/s,m/s^2)  [6]/1 -> Demux/1
  Demux/2 -> Sensor Failure (Accelerometer)/1(Sensor Input)
  Sensor Failure (Gyroscope)/1(Sensor Fault) -> Data Type Conversion2/1
  Sensor Failure (Accelerometer)/1(Sensor Fault) -> Data Type Conversion1/1
  Mux/1 -> Logical Operator/1
  Data Type Conversion2/1 -> Mux/1
  Data Type Conversion1/1 -> Mux/2
  Demux/1 -> Sensor Failure (Gyroscope)/1(Sensor Input)
  Logical Operator/1 -> Data Type Conversion4/1
  Data Type Conversion4/1 -> IMU Failure/1

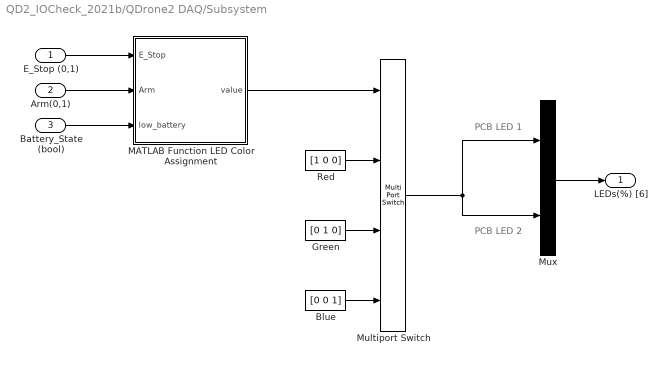
== system QD2_IOCheck_2021b/QDrone2 DAQ/Subsystem ==
  note: PCB LED 2
  note: PCB LED 1
  E_Stop (0,1) : Inport
  "Arm(0,1) " : Inport  Port=2
  Battery_State (bool) : Inport  Port=3
  Blue : Constant  Value=[0 0 1]
  Green : Constant  Value=[0 1 0]
  MATLAB Function LED Color Assignment : MATLAB Function  TreatAsAtomicUnit=on
  Multiport Switch : MultiPortSwitch
  Mux : Mux  Inputs=2
  Red : Constant  Value=[1 0 0]
  LEDs(%) [6] : Outport
  wires:
  Mux/1 -> LEDs(%) [6]/1
  Multiport Switch/1 -> Mux/1, Mux/2
  Blue/1 -> Multiport Switch/4
  Green/1 -> Multiport Switch/3
  Red/1 -> Multiport Switch/2
  Battery_State (bool)/1 -> MATLAB Function LED Color Assignment/3(low_battery)
  E_Stop (0,1)/1 -> MATLAB Function LED Color Assignment/1(E_Stop)
  "Arm(0,1) "/1 -> MATLAB Function LED Color Assignment/2(Arm)
  MATLAB Function LED Color Assignment/1(value) -> Multiport Switch/1

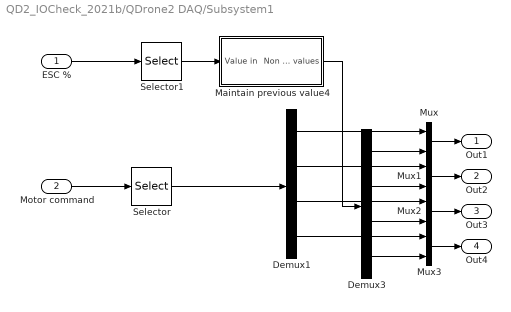
== system QD2_IOCheck_2021b/QDrone2 DAQ/Subsystem1 ==
  ESC % : Inport
  Motor command : Inport  Port=2
  Demux1 : Demux
  Demux3 : Demux
  Maintain previous value4 : Subsystem
  Mux{,1..3} (4 alike) : Mux  Inputs=2
  Selector : Selector  InputPortWidth=4  IndexOptions=Index vector (dialog)  Indices=[4 3 2 1]  OutputSizes=1
  Selector1 : Selector  InputPortWidth=4  IndexOptions=Index vector (dialog)  Indices=[4 3 2 1]  OutputSizes=1
  Out1 : Outport
  Out2 : Outport  Port=2
  Out3 : Outport  Port=3
  Out4 : Outport  Port=4
  wires:
  Motor command/1 -> Selector/1
  Demux1/2 -> Mux1/1
  Selector/1 -> Demux1/1
  Demux1/1 -> Mux/1
  Demux1/4 -> Mux3/1
  Demux1/3 -> Mux2/1
  Mux3/1 -> Out4/1
  Mux2/1 -> Out3/1
  Mux/1 -> Out1/1
  Mux1/1 -> Out2/1
  ESC %/1 -> Selector1/1
  Demux3/1 -> Mux/2
  Demux3/2 -> Mux1/2
  Demux3/3 -> Mux2/2
  Demux3/4 -> Mux3/2
  Selector1/1 -> Maintain previous value4/1(Value in)
  Maintain previous value4/1(Non 0 values) -> Demux3/1

== system QD2_IOCheck_2021b/QDrone2 DAQ/Check Battery level/Triggered Subsystem ==
  Trigger : TriggerPort  VariantControl=(inherit)
  Constant : Constant
  Out1 : Outport  InitialOutput=[0]
  wires:
  Constant/1 -> Out1/1

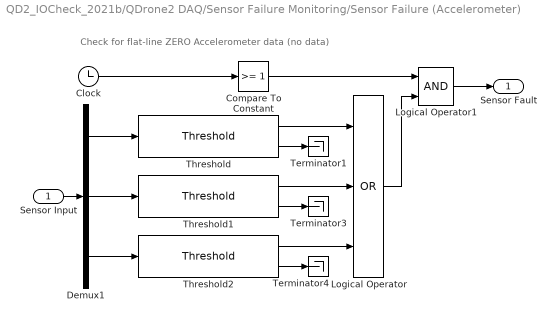
== system QD2_IOCheck_2021b/QDrone2 DAQ/Sensor Failure Monitoring/Sensor Failure (Accelerometer) ==
  note: Check for flat-line ZERO Accelerometer data (no data)
  Sensor Input : Inport
  Clock : Clock
  Compare To Constant : simulink/Logic and Bit Operations/Compare To Constant  relop=>=  const=1  OutDataTypeStr=boolean
  Demux1 : Demux  Outputs=3
  Logical Operator : Logic  Operator=OR  Inputs=3  AllPortsSameDT=off  OutDataTypeStr=boolean
  Logical Operator1 : Logic  AllPortsSameDT=off  OutDataTypeStr=boolean
  Terminator1 : Terminator
  Terminator3 : Terminator
  Terminator4 : Terminator
  Threshold : quarc_library/Discontinuities/Threshold  operator===  param_src=Specify via dialog  threshold=0  duration=1
      settings: SourceProductName=QUARC Targets
  Threshold1 : quarc_library/Discontinuities/Threshold  operator===  param_src=Specify via dialog  threshold=0  duration=1
      settings: SourceProductName=QUARC Targets
  Threshold2 : quarc_library/Discontinuities/Threshold  operator===  param_src=Specify via dialog  threshold=0  duration=1
      settings: SourceProductName=QUARC Targets
  Sensor Fault : Outport  VectorParamsAs1DForOutWhenUnconnected=off
  wires:
  Clock/1 -> Compare To Constant/1
  Threshold/1 -> Logical Operator/1
  Threshold1/1 -> Logical Operator/2
  Compare To Constant/1 -> Logical Operator1/1
  Logical Operator1/1 -> Sensor Fault/1
  Sensor Input/1 -> Demux1/1
  Threshold2/2 -> Terminator4/1
  Threshold2/1 -> Logical Operator/3
  Demux1/1 -> Threshold/1
  Demux1/3 -> Threshold2/1
  Demux1/2 -> Threshold1/1
  Logical Operator/1 -> Logical Operator1/2
  Threshold1/2 -> Terminator3/1
  Threshold/2 -> Terminator1/1

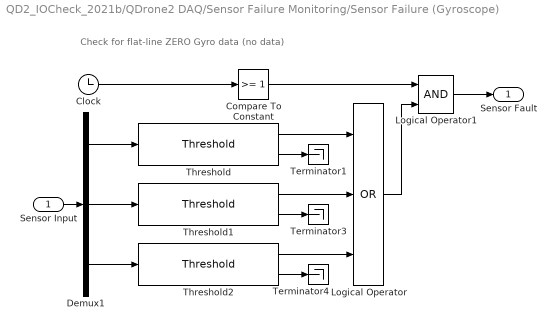
== system QD2_IOCheck_2021b/QDrone2 DAQ/Sensor Failure Monitoring/Sensor Failure (Gyroscope) ==
  note: Check for flat-line ZERO Gyro data (no data)
  Sensor Input : Inport
  Clock : Clock
  Compare To Constant : simulink/Logic and Bit Operations/Compare To Constant  relop=>=  const=1  OutDataTypeStr=boolean
  Demux1 : Demux  Outputs=3
  Logical Operator : Logic  Operator=OR  Inputs=3  AllPortsSameDT=off  OutDataTypeStr=boolean
  Logical Operator1 : Logic  AllPortsSameDT=off  OutDataTypeStr=boolean
  Terminator1 : Terminator
  Terminator3 : Terminator
  Terminator4 : Terminator
  Threshold : quarc_library/Discontinuities/Threshold  operator===  param_src=Specify via dialog  threshold=0  duration=1
      settings: SourceProductName=QUARC Targets
  Threshold1 : quarc_library/Discontinuities/Threshold  operator===  param_src=Specify via dialog  threshold=0  duration=1
      settings: SourceProductName=QUARC Targets
  Threshold2 : quarc_library/Discontinuities/Threshold  operator===  param_src=Specify via dialog  threshold=0  duration=1
      settings: SourceProductName=QUARC Targets
  Sensor Fault : Outport  VectorParamsAs1DForOutWhenUnconnected=off
  wires:
  Threshold/2 -> Terminator1/1
  Threshold1/2 -> Terminator3/1
  Logical Operator/1 -> Logical Operator1/2
  Demux1/2 -> Threshold1/1
  Demux1/3 -> Threshold2/1
  Demux1/1 -> Threshold/1
  Threshold2/1 -> Logical Operator/3
  Threshold2/2 -> Terminator4/1
  Sensor Input/1 -> Demux1/1
  Logical Operator1/1 -> Sensor Fault/1
  Compare To Constant/1 -> Logical Operator1/1
  Threshold1/1 -> Logical Operator/2
  Threshold/1 -> Logical Operator/1
  Clock/1 -> Compare To Constant/1

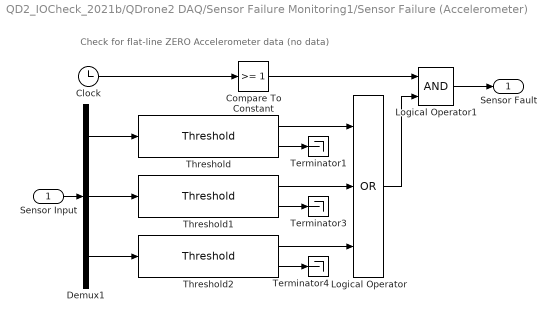
== system QD2_IOCheck_2021b/QDrone2 DAQ/Sensor Failure Monitoring1/Sensor Failure (Accelerometer) ==
  note: Check for flat-line ZERO Accelerometer data (no data)
  Sensor Input : Inport
  Clock : Clock
  Compare To Constant : simulink/Logic and Bit Operations/Compare To Constant  relop=>=  const=1  OutDataTypeStr=boolean
  Demux1 : Demux  Outputs=3
  Logical Operator : Logic  Operator=OR  Inputs=3  AllPortsSameDT=off  OutDataTypeStr=boolean
  Logical Operator1 : Logic  AllPortsSameDT=off  OutDataTypeStr=boolean
  Terminator1 : Terminator
  Terminator3 : Terminator
  Terminator4 : Terminator
  Threshold : quarc_library/Discontinuities/Threshold  operator===  param_src=Specify via dialog  threshold=0  duration=1
      settings: SourceProductName=QUARC Targets
  Threshold1 : quarc_library/Discontinuities/Threshold  operator===  param_src=Specify via dialog  threshold=0  duration=1
      settings: SourceProductName=QUARC Targets
  Threshold2 : quarc_library/Discontinuities/Threshold  operator===  param_src=Specify via dialog  threshold=0  duration=1
      settings: SourceProductName=QUARC Targets
  Sensor Fault : Outport  VectorParamsAs1DForOutWhenUnconnected=off
  wires:
  Threshold/2 -> Terminator1/1
  Threshold1/2 -> Terminator3/1
  Logical Operator/1 -> Logical Operator1/2
  Demux1/2 -> Threshold1/1
  Demux1/3 -> Threshold2/1
  Demux1/1 -> Threshold/1
  Threshold2/1 -> Logical Operator/3
  Threshold2/2 -> Terminator4/1
  Sensor Input/1 -> Demux1/1
  Logical Operator1/1 -> Sensor Fault/1
  Compare To Constant/1 -> Logical Operator1/1
  Threshold1/1 -> Logical Operator/2
  Threshold/1 -> Logical Operator/1
  Clock/1 -> Compare To Constant/1

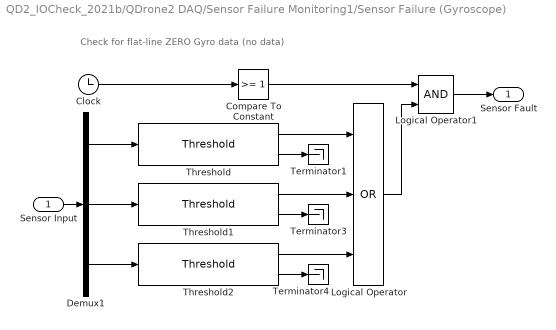
== system QD2_IOCheck_2021b/QDrone2 DAQ/Sensor Failure Monitoring1/Sensor Failure (Gyroscope) ==
  note: Check for flat-line ZERO Gyro data (no data)
  Sensor Input : Inport
  Clock : Clock
  Compare To Constant : simulink/Logic and Bit Operations/Compare To Constant  relop=>=  const=1  OutDataTypeStr=boolean
  Demux1 : Demux  Outputs=3
  Logical Operator : Logic  Operator=OR  Inputs=3  AllPortsSameDT=off  OutDataTypeStr=boolean
  Logical Operator1 : Logic  AllPortsSameDT=off  OutDataTypeStr=boolean
  Terminator1 : Terminator
  Terminator3 : Terminator
  Terminator4 : Terminator
  Threshold : quarc_library/Discontinuities/Threshold  operator===  param_src=Specify via dialog  threshold=0  duration=1
      settings: SourceProductName=QUARC Targets
  Threshold1 : quarc_library/Discontinuities/Threshold  operator===  param_src=Specify via dialog  threshold=0  duration=1
      settings: SourceProductName=QUARC Targets
  Threshold2 : quarc_library/Discontinuities/Threshold  operator===  param_src=Specify via dialog  threshold=0  duration=1
      settings: SourceProductName=QUARC Targets
  Sensor Fault : Outport  VectorParamsAs1DForOutWhenUnconnected=off
  wires:
  Clock/1 -> Compare To Constant/1
  Threshold/1 -> Logical Operator/1
  Threshold1/1 -> Logical Operator/2
  Compare To Constant/1 -> Logical Operator1/1
  Logical Operator1/1 -> Sensor Fault/1
  Sensor Input/1 -> Demux1/1
  Threshold2/2 -> Terminator4/1
  Threshold2/1 -> Logical Operator/3
  Demux1/1 -> Threshold/1
  Demux1/3 -> Threshold2/1
  Demux1/2 -> Threshold1/1
  Logical Operator/1 -> Logical Operator1/2
  Threshold1/2 -> Terminator3/1
  Threshold/2 -> Terminator1/1

== system QD2_IOCheck_2021b/QDrone2 DAQ/Subsystem1/Maintain previous value4 ==
  Value in : Inport
  Memory : Memory
  Switch : Switch  Criteria=u2 ~= 0
  Non 0 values : Outport
  wires:
  Value in/1 -> Switch/1, Switch/2
  Switch/1 -> Memory/1, Non 0 values/1
  Memory/1 -> Switch/3

== matlab function QD2_IOCheck_2021b/QDrone2 DAQ/Subsystem/MATLAB Function LED Color Assignment ==
  data: E_Stop input; Arm input; value output; low_battery input
function value = fcn(E_Stop, Arm, low_battery)

if low_battery == 1|| E_Stop ==1
    value = 1;
elseif Arm == 1 & E_Stop ==0
    value = 2;
elseif Arm == 0 && E_Stop == 0 
    value = 3;
else 
    value = 3;
end

== matlab function QD2_IOCheck_2021b/QDrone2 DAQ/MotorCMD_FSM ==
  data: Arm_Signal input; E_Stop input; ESC_cmd output; Motor_State output; Model_Time input; Motor_State input
function [ESC_cmd,Motor_State]= fcn(Arm_Signal,E_Stop,Model_Time, Motor_State)

persistent state ESC_CMD 

%  Initialize motor state at the start of the model
if isempty(state)
    state = 2;
    ESC_CMD = zeros(1,4);
end 

% ESC Numbers w.r.t motor positions on QDrone: 
%         FRONT
%       4(3)       2(1)
% 
%       3(2)       1(0)
%          BACK  


% ============ Motor programing state machine ============ 

% State machine transitions: 

% Motor configuration state: 
if E_Stop == 0 && state ~= 9
    % Start with the motors in an idle state    
    if state == 2 && Model_Time > 0 && Model_Time <= 1  
        if Arm_Signal == 1
            % Error state, you started the model while the QDrone was armed
            state = 9;
        end 
           
    elseif state ==2  && Model_Time > 1 && Model_Time <= 2
        % Enter motor Low Frequency state:
        state = 1;
        
    elseif state ==1  && Model_Time > 2 && Model_Time <= 2.5
        % Set motor orientation
        state = 0;
        
    elseif state == 0 && Model_Time > 2.5    
        % Enter motor idle state: 
        state = 2; 

    elseif Motor_State ==2 && Arm_Signal == 1 
        % Enter arm state 
        state = 3;

    elseif Motor_State ==3 && Arm_Signal ==0 
        % Return to idle state 
        state = 2; 
    end 
    
elseif E_Stop ==1 
    % You've entered emergency state, disarm QDrone2!
    state = 9; 
end 


% State Machine commands: 
switch state 
    
    % ESC orientation set:
    case 0
        % for all drones
        ESC_CMD = [20,21,21,20];
        %for 1st R&D Drone 
        % ESC_CMD = [0,0,0,0];
    
    % Motor Low Frequency Beep:
    case 1
        ESC_CMD = [1,1,1,1];
    
    % Enter motor stop state: 
    case 2
        ESC_CMD = [0,0,0,0];
    
    % Motors in Arm State:
    case 3
        ESC_CMD = [48,48,48,48];
        
    % Same as state 2 but used as an Error State to stop motor cmd:
    case 9
        ESC_CMD = [0,0,0,0];
        
end 
    


Motor_State = state;
ESC_cmd = ESC_CMD;

Motor_State, ESC_cmd;

== matlab function QD2_IOCheck_2021b/QDrone2 DAQ/roll and pitch approximation from accelerometer ==
  data: roll_acc output; pitch_acc output; acc_body input
function [roll_acc, pitch_acc]   = fcn(acc_body)
%#eml
n = norm(acc_body,2);
if n>eps
    acc_body = acc_body/n; 
else
    acc_body = [0 0 1]';
end

roll_acc = atan2(acc_body(2),acc_body(3));
pitch_acc = atan2( -acc_body(1), acc_body(2)*sin(roll_acc)+acc_body(3)*cos(roll_acc));

== matlab function QD2_IOCheck_2021b/QDrone2 DAQ/roll and pitch approximation from accelerometer1 ==
  data: roll_acc output; pitch_acc output; acc_body input
function [roll_acc, pitch_acc]   = fcn(acc_body)
%#eml
n = norm(acc_body,2);
if n>eps
    acc_body = acc_body/n; 
else
    acc_body = [0 0 1]';
end

roll_acc = atan2(acc_body(2),acc_body(3));
pitch_acc = atan2( -acc_body(1), acc_body(2)*sin(roll_acc)+acc_body(3)*cos(roll_acc));
